simulink model "System"  (R2023a)
settings: Solver=VariableStepAuto  StartTime=0.0  StopTime=10.0  RelTol=1e-3
settings Model: Creator=HP Elitebook  LastModifiedBy=HP Elitebook
settings DataIOCC: ReturnWorkspaceOutputs=off

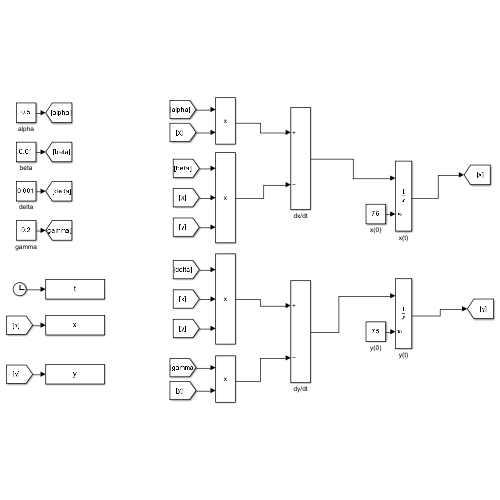
[thumbnail: Simulink's stored preview of the top-level diagram]
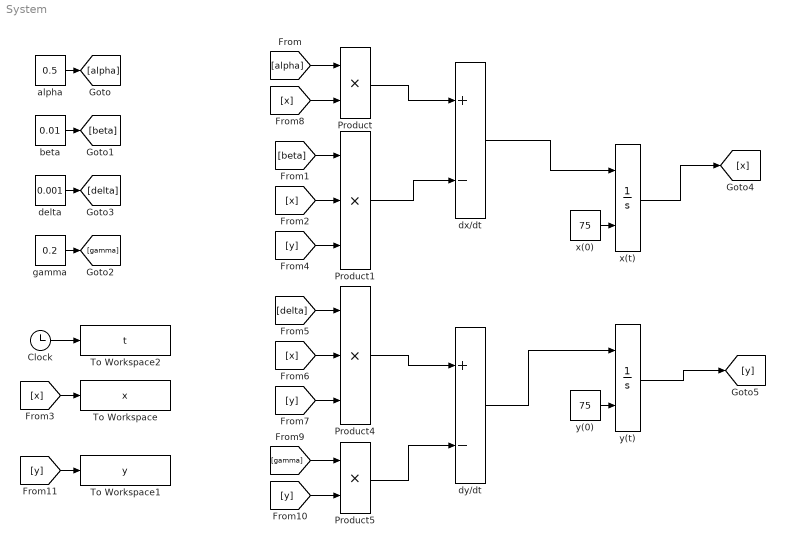
== system System ==
  Clock : Clock
  Product : Product
  Product1 : Product  Inputs=3
  Product4 : Product  Inputs=3
  Product5 : Product
  To Workspace : ToWorkspace  VariableName=x  SampleTime=-1
  To Workspace1 : ToWorkspace  VariableName=y  SampleTime=-1
  To Workspace2 : ToWorkspace  VariableName=t  SampleTime=-1
  alpha : Constant  Value=0.5
  beta : Constant  Value=0.01
  delta : Constant  Value=0.001
  dx/dt : Sum  Inputs=+-
  dy/dt : Sum  Inputs=+-
  gamma : Constant  Value=0.2
  x(0) : Constant  Value=75
  x(t) : Integrator  InitialConditionSource=external
  y(0) : Constant  Value=75
  y(t) : Integrator  InitialConditionSource=external
  wires:
  alpha/1 -> [alpha]
  [alpha] -> Product/1
  beta/1 -> [beta]
  gamma/1 -> [gamma]
  delta/1 -> [delta]
  [beta] -> Product1/1
  [x] -> Product1/2
  [y] -> Product1/3
  [y] -> Product4/3
  [delta] -> Product4/1
  [x] -> Product4/2
  [x] -> Product/2
  [gamma] -> Product5/1
  [y] -> Product5/2
  x(0)/1 -> x(t)/2
  y(0)/1 -> y(t)/2
  Product/1 -> dx/dt/1
  Product1/1 -> dx/dt/2
  Product4/1 -> dy/dt/1
  Product5/1 -> dy/dt/2
  dy/dt/1 -> y(t)/1
  dx/dt/1 -> x(t)/1
  x(t)/1 -> [x]
  y(t)/1 -> [y]
  Clock/1 -> To Workspace2/1
  [y] -> To Workspace1/1
  [x] -> To Workspace/1
